simulink model "Motor_Simulink"  (R2015a)
settings: Solver=ode45  StartTime=0.0  StopTime=10.0  RelTol=1e-3
values from neighbouring files (symbols this model uses):
  b = 5    [Prac_6_Solution.m]
  J = 10    [Prac_6_Solution.m]
  K = 1    [Prac_6_Solution.m]
  L = 0.01    [Prac_6_Solution.m]
  R = 5    [Prac_6_Solution.m]
settings Model: Creator=DELL  LastModifiedBy=DELL

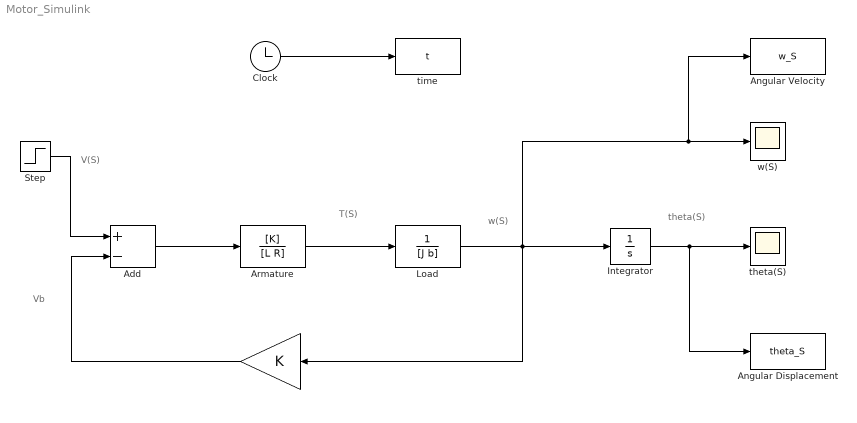
== system Motor_Simulink ==
  note: theta(S)
  note: w(S)
  note: T(S)
  note: Vb
  note: V(S)
  " " : Gain  Gain=K
  Add : Sum  Inputs=+-
  Angular Displacement : ToWorkspace  VariableName=theta_S  SampleTime=-1
  Angular Velocity : ToWorkspace  VariableName=w_S  SampleTime=-1
  Armature : TransferFcn  Numerator=[K]  Denominator=[L R]
  Clock : Clock
  Integrator : Integrator
  Load : TransferFcn  Denominator=[J b]
  Step : Step  SampleTime=0
  theta(S) : Scope
  time : ToWorkspace  VariableName=t  SampleTime=-1
  w(S) : Scope
  wires:
  Armature/1 -> Load/1
  Load/1 -> Angular Velocity/1, w(S)/1, Integrator/1, " "/1
  Add/1 -> Armature/1
  " "/1 -> Add/2
  Step/1 -> Add/1
  Integrator/1 -> theta(S)/1, Angular Displacement/1
  Clock/1 -> time/1
